simulink model "linear_model_with_disturbance"  (R2025a)
settings: Solver=VariableStepAuto  StartTime=0.0  StopTime=100.0  RelTol=1e-3
libraries: slpidlib x1
settings Model: Creator=Kush  LastModifiedBy=Kush

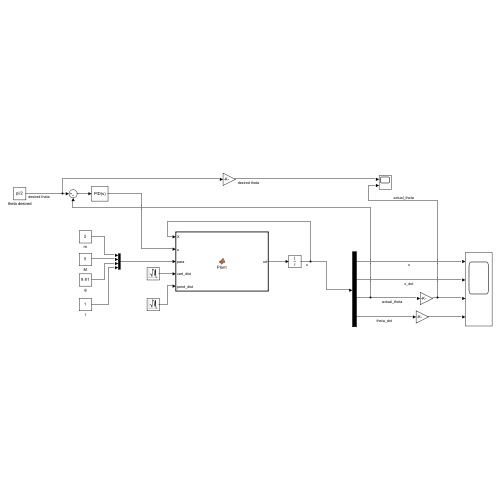
[thumbnail: Simulink's stored preview of the top-level diagram]
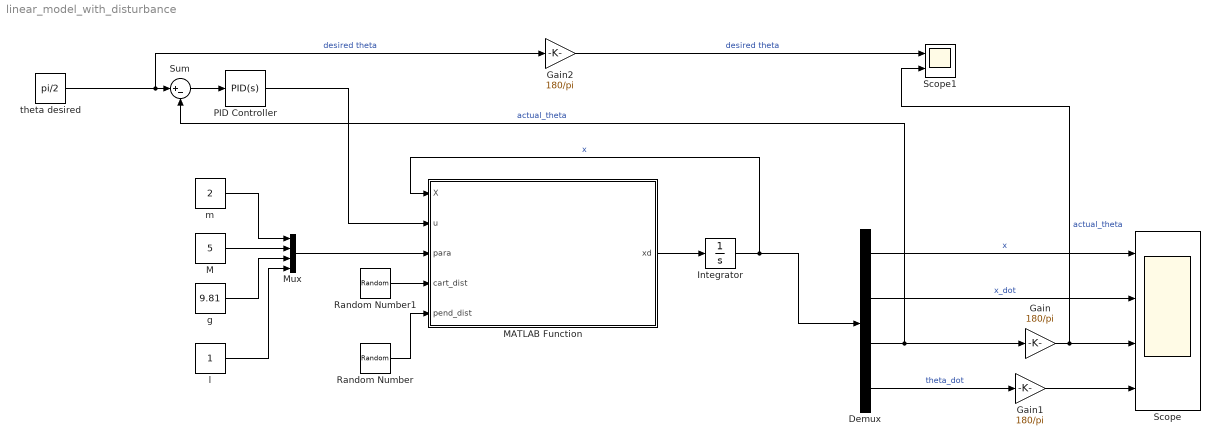
== system linear_model_with_disturbance ==
  Demux : Demux
  Gain : Gain  Gain=180/pi
  Gain1 : Gain  Gain=180/pi
  Gain2 : Gain  Gain=180/pi
  Integrator : Integrator
  M : Constant  Value=5
  MATLAB Function : MATLAB Function  TreatAsAtomicUnit=on
  Mux : Mux
  PID Controller : slpidlib/PID Controller  Controller=PID  Form=Parallel  TimeDomain=Continuous-time  UseExternalTs=off  SampleTime=-1  IntegratorMethod=Forward Euler  FilterMethod=Forward Euler  ControllerParametersSource=internal  P=-950.33453317524  I=-1818.34018122408  UseKiTs=off  D=-108.274913194782  UseExternalDerivativeSource=off  N=329.421305606589  UseFilter=on  TunerSelectOption=Transfer Function Based (PID Tuner App)  InitialConditionSource=internal  InitialConditionForIntegrator=0  InitialConditionForFilter=0  DifferentiatorICPrevScaledInput=0  ExternalReset=none  TrackingMode=off  Kt=1  LimitOutput=off  SatLimitsSource=internal  UpperSaturationLimit=inf  LowerSaturationLimit=-inf  LinearizeAsGain=on  AntiWindupMode=none  Kb=1  LimitIntegrator=off  UpperIntegratorSaturationLimit=inf  LowerIntegratorSaturationLimit=-inf  POutMin=[]  POutMax=[]  IOutMin=[]  IOutMax=[]  DOutMin=[]  DOutMax=[]  NOutMin=[]  NOutMax=[]  SumOutMin=[]  SumOutMax=[]  SaturationOutMin=[]  SaturationOutMax=[]  PParamMin=[]  PParamMax=[]  IParamMin=[]  IParamMax=[]  DParamMin=[]  DParamMax=[]  NParamMin=[]  NParamMax=[]  KbParamMin=[]  KbParamMax=[]  KtParamMin=[]  KtParamMax=[]  KbOutMin=[]  KbOutMax=[]  KtOutMin=[]  KtOutMax=[]  IntegratorOutMin=[]  IntegratorOutMax=[]  FilterOutMin=[]  FilterOutMax=[]  SumI1OutMin=[]  SumI1OutMax=[]  SumI2OutMin=[]  SumI2OutMax=[]  SumI3OutMin=[]  SumI3OutMax=[]  SumI4OutMin=[]  SumI4OutMax=[]  SumDOutMin=[]  SumDOutMax=[]  DifferentiatorOutMin=[]  DifferentiatorOutMax=[]  FilterDiffOutCoefMin=[]  FilterDiffOutCoefMax=[]  ReciprocalOutMin=[]  ReciprocalOutMax=[]  SumDenOutMin=[]  SumDenOutMax=[]  SumNumOutMin=[]  SumNumOutMax=[]  DivideOutMin=[]  DivideOutMax=[]  UdiffTsProdOutMin=[]  UdiffTsProdOutMax=[]  NTsProdOutMin=[]  NTsProdOutMax=[]  UintegralTsProdOutMin=[]  UintegralTsProdOutMax=[]  UngainTsProdOutMin=[]  UngainTsProdOutMax=[]  ClampingZeroOutDataTypeStr=Inherit: Inherit via back propagation  ClampingZeroOutMin=[]  ClampingZeroOutMax=[]  FilterDenConstantOutDataTypeStr=Inherit: Inherit via back propagation  FilterDenConstantOutMin=[]  FilterDenConstantOutMax=[]  PCopyOutDataTypeStr=Inherit: Inherit via back propagation  PCopyOutMin=[]  PCopyOutMax=[]  NCopyOutDataTypeStr=Inherit: Inherit via back propagation  NCopyOutMin=[]  NCopyOutMax=[]  IntegratorContinuousStateAttributes=''  IntegratorStateMustResolveToSignalObject=off  IntegratorRTWStateStorageClass=Auto  FilterContinuousStateAttributes=''  FilterStateMustResolveToSignalObject=off  FilterRTWStateStorageClass=Auto  ParallelPVariant=InternalParameters  IdealPVariant=Disabled  IVariant=InternalParameters  DVariant=InternalParameters  IntegratorVariant=Continuous  SatVariant=Disabled  AWVariant=Passthrough  PCopyVariant=Disabled  TRVariant=Disabled  FdbkBlocksVariant=Forward  IdealPFdbkVariant=Disabled  SatFdbkVariant=Disabled  DerivativeFilterVariant=ContFilter  NVariant=InternalParameters  NCopyVariant=Disabled  FilterICVariant=InternalICsFilter  IntegratorICVariant=InternalICs  ExternalResetVariant=Disabled  TRSumVariant=Passthrough  SumFdbkVariant=Disabled  SumVariant=Sum_PID  TsampFilterVariant=InternalTs  TsampNgainVariant=Passthrough  TsampIntegralVariant=Disabled_SignalSpec  ExternalSaturationOutDataTypeStr=Inherit: Same as second input  DerivativeSourceVariant=ErrorSignal  PreIntVariant=InternalPreInt
  Random Number : RandomNumber  SampleTime=0.1
  Random Number1 : RandomNumber  SampleTime=0.1
  Scope : Scope  NumInputPorts=4
      settings: SampleTime=0.01  ActiveDisplayYMinimum=-174247.6815700311  ActiveDisplayYMaximum=19360.85350778123
  Scope1 : Scope  NumInputPorts=2
      settings: SampleTime=0.01  ActiveDisplayYMinimum=47.2838250048203  ActiveDisplayYMaximum=354.01849546420749
  Sum : Sum  Inputs=|+-
  g : Constant  Value=9.81
  l : Constant
  m : Constant  Value=2
  theta desired : Constant  Value=pi/2
  wires:
  m/1 -> Mux/1
  M/1 -> Mux/2
  g/1 -> Mux/3
  l/1 -> Mux/4
  Mux/1 -> MATLAB Function/3(para)
  Random Number/1 -> MATLAB Function/5(pend_dist)
  Random Number1/1 -> MATLAB Function/4(cart_dist)
  MATLAB Function/1(xd) -> Integrator/1
  Integrator/1 -> MATLAB Function/1(X), Demux/1  "x"
  Demux/1 -> Scope/1  "x"
  Demux/2 -> Scope/2  "x_dot"
  Demux/4 -> Gain1/1  "theta_dot"
  PID Controller/1 -> MATLAB Function/2(u)
  theta desired/1 -> Gain2/1, Sum/1  "desired theta"
  Gain1/1 -> Scope/4
  Demux/3 -> Gain/1, Sum/2  "actual_theta"
  Gain/1 -> Scope1/2, Scope/3  "actual_theta"
  Sum/1 -> PID Controller/1
  Gain2/1 -> Scope1/1  "desired theta"

== matlab function linear_model_with_disturbance/MATLAB Function ==
  data: X input size=[4 1]; u input size=[1 1]; xd output size=[4 1]; para input size=[4 1]; cart_dist input size=[1 1]; pend_dist input size=[1 1]
function xd = Plant(X,u,para,cart_dist,pend_dist)
m = para(1);
M = para(2);
g = para(3);
l = para(4);

x =         X(1);
x_dot =     X(2);
theta =     X(3);
theta_dot = X(4);

den = 4*M +m;
u_final = u + cart_dist ;
theta_final = theta + pend_dist;

x_ddot = 4*u_final/den + 3*m*g*theta_final/den;
theta_ddot = -6*u_final/(den*l) -6*(M+m)*theta_final*g/(den*l);

xd = [x_dot;x_ddot;theta_dot;theta_ddot];
